simulink model "ForceMomentCBAgent"  (Simulink 7.1)
settings: Solver=ode45  SolverMode=SingleTasking  StartTime=0.0  StopTime=10.0  RelTol=1e-3  AbsTol=1e-6
settings Model: Creator=The MathWorks Inc.  LastModifiedBy=suarezjl  ExtModeTrigMode=oneshot  ExtModeArmWhenConnect=off  ExtModeAutoUpdateStatusClock=off
settings DataIOCC: LimitDataPoints=off  SignalLoggingName=logsOut
settings OptimizationCC: BooleanDataType=off  InlineInvariantSignals=on
settings DebuggingCC: SaveWithParameterizedLinksMsg=none  CheckExecutionContextPreStartOutputMsg=on  CheckExecutionContextRuntimeOutputMsg=on  SignalResolutionControl=TryResolveAllWithWarning  SolverPrmCheckMsg=none  MultiTaskDSMMsg=warning  MultiTaskCondExecSysMsg=none  IntegerOverflowMsg=none  StrictBusMsg=None
settings HardwareCC: TargetUnknown=on
settings ModelReferenceCC: UpdateModelReferenceTargets=IfOutOfDate
settings RTWCC: IncludeERTFirstTime=on
settings GRTTargetCC: TargetFcnLib=ansi_tfl_tmw.mat

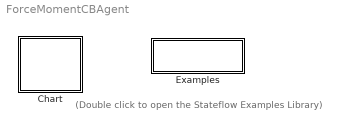
== system ForceMomentCBAgent ==
  note: (Double click to open the
      | Stateflow Examples Library)
  Chart : Stateflow chart
  Examples : Subsystem
      settings: OpenFcn=sf('Private','sf_examples')
      mask Display: disp('Examples')

== system ForceMomentCBAgent/Examples ==

== stateflow chart Chart ==
  state Initialize
    \\Octavia\ISACControlBasisModule\LeftModule\Arm\ArmController.DoHomingRoutine()
    \\Octavia\ISACControlBasisModule\RightModule\Arm\ArmController.DoHomingRoutine()
    \\Octavia\ISACControlBasisModule\ForceMomentCB\StateMachine.Wait(5000)
    \\Octavia\ISACControlBasisModule\LeftModule\Arm\InverseKinematics.Initialize()
    \\Octavia\ISACControlBasisModule\RightModule\Arm\InverseKinematics.Initialize()
  state ControlBasis
    \\Octavia\ISACControlBasisModule\LeftModule\Arm\ArmController.Move()
    \\Octavia\ISACControlBasisModule\RightModule\Arm\ArmController.Move()
    \\Octavia\ISACControlBasisModule\ForceMomentCB\ForceMomentCB.ComputeControlBasis()
  state Stop
    \\Octavia\ISACControlBasisModule\LeftModule\Arm\ArmController.DoHomingRoutine()
    \\Octavia\ISACControlBasisModule\RightModule\Arm\ArmController.DoHomingRoutine()
    \\Octavia\ISACControlBasisModule\ForceMomentCB\StateMachine.Wait(5000)
  state StartStateMachines
    \\Octavia\ISACControlBasisModule\LeftModule\ForceSensor\StateMachine.LoadSM()
    \\Octavia\ISACControlBasisModule\RightModule\ForceSensor\StateMachine.LoadSM()
    \\Octavia\ISACControlBasisModule\LeftModule\ForceSensor\StateMachine.Start()
    \\Octavia\ISACControlBasisModule\RightModule\ForceSensor\StateMachine.Start()
    \\Octavia\ISACControlBasisModule\VirtualContact\StateMachine.LoadSM()
    \\Octavia\ISACControlBasisModule\VirtualContact\StateMachine.Start()
  state Close
    \\Octavia\ISACControlBasisModule\LeftModule\Arm\ArmController.Close()
    \\Octavia\ISACControlBasisModule\RightModule\Arm\ArmController.Close()
    \\Octavia\ISACControlBasisModule\ForceMomentCB\StateMachine.Wait(5000)
  (default) -> Initialize : Start
  Initialize -> StartStateMachines : Always
  ControlBasis -> ControlBasis [order 1] : Default
  ControlBasis -> Stop [order 3] : Signal="Stop"
  StartStateMachines -> ControlBasis : Always
  Stop -> Close : Signal="Close"
  ControlBasis -> Close [order 2] : Signal="Close"
